simulink library "Power_Electric2Motor"  (R2020a)
settings: Solver=VariableStepAuto  StartTime=0.0  StopTime=10.0  RelTol=1e-3
undefined symbols (not defined in the file): Powertrain, ShaftF, ShaftR
libraries: Power_Components x3, fl_lib x2, sm_lib x1, Cooling_2_Motor x1
Description:
  | Component of Simscape Vehicle Templates Library
  | 
  | Copyright 2018-2020 The MathWorks, Inc.
settings Model: Creator=smiller  LastModifiedBy=smiller
settings DataIOCC: ReturnWorkspaceOutputs=off
settings DebuggingCC: ArithmeticOperatorsInVariantConditions=warning
settings SFSimCC: CustomCodeUndefinedFunction=UseInterfaceOnly

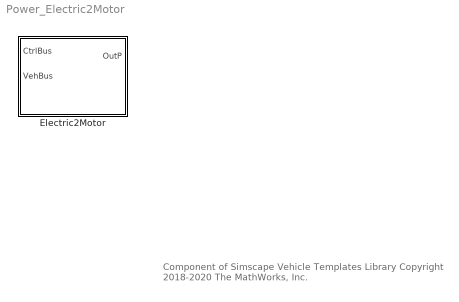
== system Power_Electric2Motor ==
  note: Component of Simscape Vehicle Templates Library
      | Copyright 2018-2020 The MathWorks, Inc.
  Electric2Motor : Subsystem  VariantControl=ElectricTwoMotor  mask(Electric Propulsion with Two Motors){Power=Powertrain.Power, InitTriggerDropdown=0}
      mask prompts: Power "Power 2 Motor (Structure)"; InitTriggerDropdown "Initialization Trigger Dropdown"
      mask help: Two electric motors with optional cooling system. Physical connections for the three motor shafts are in bus Shafts.
      mask init:
      | curblk = gcb;
      | 
      | % Trigger Mask Initialization for 
      | % variant subsystems below this level
      | sm_car_lib_maskInitTrigger(curblk)
      mask TypeOptions InitTriggerDropdown: 0 | 1
      mask Display: image('sm_car_vehicle_power_e2motor_IMAGE.png');

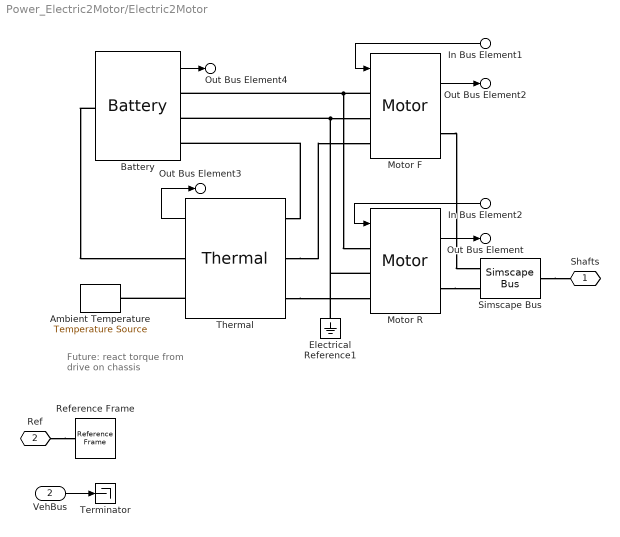
== system Power_Electric2Motor/Electric2Motor ==
  note: Future:
      | react torque
      | from drive
      | on chassis
  In Bus Element1 : Inport  PortName=CtrlBus  Element=MMotorFDemand
  In Bus Element2 : Inport  PortName=CtrlBus  Element=MMotorRDemand
  VehBus : Inport  Port=2
  Ambient Temperature : fl_lib/Thermal/Thermal Sources/Temperature Source  temperature=Power.TAmbient.Value K
  Battery : Power_Components/Battery  SystemSampleTime=-1  Latency=0  AutoFrameSizeCalculation=off
  Electrical Reference1 : fl_lib/Electrical/Electrical Elements/Electrical Reference
  Motor F : Power_Components/Motor  Motor=Power.MotorF
  Motor R : Power_Components/Motor  Motor=Power.MotorR
  Reference Frame : sm_lib/Frames and Transforms/Reference Frame
  Simscape Bus : SimscapeBus  HierarchyStrings=ShaftF;ShaftR
  Terminator : Terminator
  Thermal : Cooling_2_Motor/Thermal  VariantControl=Variant1  VariantLabel=Power.Cooling.class.Value  InitTriggerDropdown=0
      settings: AttributesFormatString=%<ActiveVariant>
  Shafts : PMIOPort  Side=Left
  Ref : PMIOPort  Port=2  Side=Right
  Out Bus Element : Outport  VectorParamsAs1DForOutWhenUnconnected=off  PortName=OutP  Element=MotorR
  Out Bus Element2 : Outport  VectorParamsAs1DForOutWhenUnconnected=off  PortName=OutP  Element=MotorF
  Out Bus Element3 : Outport  VectorParamsAs1DForOutWhenUnconnected=off  PortName=OutP  Element=Thermal
  Out Bus Element4 : Outport  VectorParamsAs1DForOutWhenUnconnected=off  PortName=OutP  Element=Battery
  wires:
  Motor R/1 -> Out Bus Element/1
  In Bus Element2/1 -> Motor R/1
  In Bus Element1/1 -> Motor F/1
  Motor F/1 -> Out Bus Element2/1
  Thermal/1 -> Out Bus Element3/1
  VehBus/1 -> Terminator/1
  Battery/1 -> Out Bus Element4/1
  connections:
  Motor F/LConn1 -- Battery/RConn1 -- Motor R/LConn1
  Motor R/LConn2 -- Electrical Reference1/LConn1 -- Battery/RConn2 -- Motor F/LConn2
  Motor F/RConn1 -- Simscape Bus/LConn1
  Simscape Bus/RConn1 -- Shafts/RConn1
  Ref/RConn1 -- Reference Frame/RConn1
  Motor R/RConn1 -- Simscape Bus/LConn2
  Thermal/LConn1 -- Battery/RConn3
  Thermal/LConn2 -- Motor F/LConn3
  Thermal/LConn3 -- Motor R/LConn3
  Thermal/RConn2 -- Ambient Temperature/LConn1
  Battery/LConn1 -- Thermal/RConn1
